simulink model "UUV_animation"  (Simulink 7.8)
settings: Solver=ode45  StartTime=0.0  StopTime=1000  RelTol=1e-3
undefined symbols (not defined in the file or in its folder): drawUUV
libraries: simulink x1
settings Model: Creator=beard  LastModifiedBy=ecestudent
settings OptimizationCC: InitFltsAndDblsToZero=on
settings DebuggingCC: FcnCallInpInsideContextMsg=Use local settings  StrictBusMsg=Warning

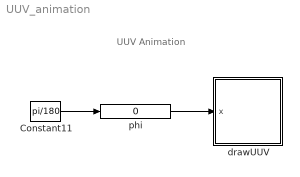
== system UUV_animation ==
  note: UUV Animation
  Constant11 : Constant  Value=pi/180
  drawUUV : Subsystem
      mask init:
      | % drawing parameters
      | MajorAxis = 10;
      | MinorAxis = 6;
      | C_M = [0;-4];
      mask Display: image(imread('tv.jpg'))
  phi : simulink/Math Operations/Slider Gain  low=-180  gain=0  high=180
  wires:
  phi/1 -> drawUUV/1(x)
  Constant11/1 -> phi/1

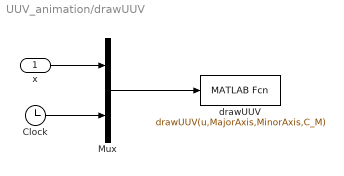
== system UUV_animation/drawUUV ==
  x : Inport
  Clock : Clock
  Mux : Mux  Inputs=2
  drawUUV : MATLABFcn  MATLABFcn=drawUUV(u,MajorAxis,MinorAxis,C_M)  OutputDimensions=0  SampleTime=0.1
  wires:
  Mux/1 -> drawUUV/1
  x/1 -> Mux/1
  Clock/1 -> Mux/2
